simulink model "Kalman_modelling"  (R2020b)
settings: Solver=VariableStepAuto  StartTime=0.0  StopTime=10.0  RelTol=1e-3
values from neighbouring files (symbols this model uses):
  A_d = sys_d.A    [sample_ss.m]
  B_d = sys_d.B    [sample_ss.m]
  C_d = sys_d.C    [sample_ss.m]
  dT = 0.05    [sample_ss.m]
  G = eye(6)    [sample_ss.m]
  Qcov = diag(0.15*ones(1,size(A_m,1)))    [sample_ss.m]
  Rcov = diag(0.05*ones(1,size(A_m,1)))    [sample_ss.m]
undefined symbols (not defined in the file or in its folder): L
libraries: simulink x2
settings Model: Creator=surya  LastModifiedBy=surya

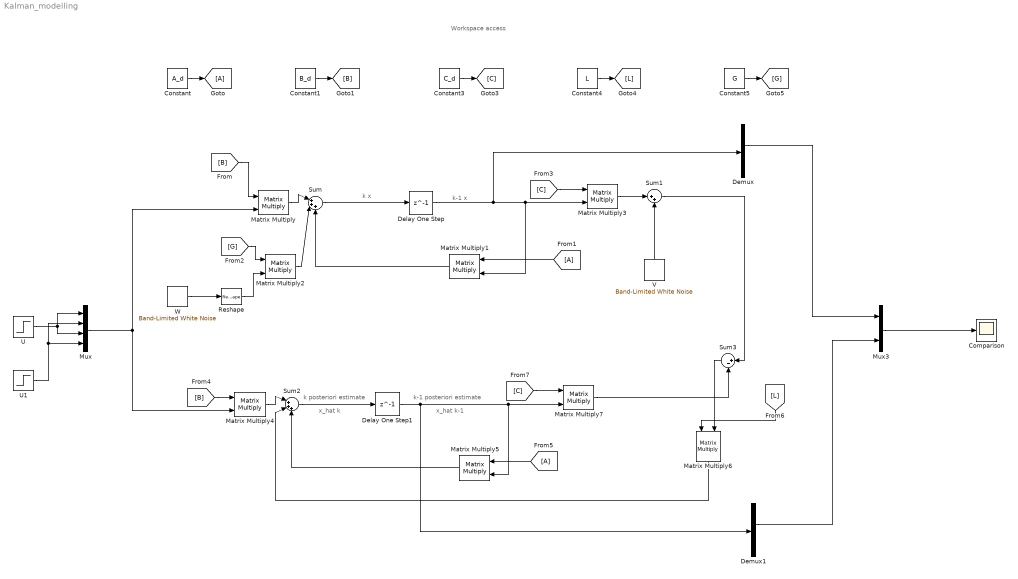
== system Kalman_modelling ==
  note: Workspace access
  note: x_hat k
  note: k x
  note: k-1 x
  note: k-1 posteriori estimate
  note: k posteriori estimate
  note: x_hat k-1
  Comparison : Scope
  Constant : Constant  Value=A_d
  Constant1 : Constant  Value=B_d
  Constant3 : Constant  Value=C_d
  Constant4 : Constant  Value=L
  Constant5 : Constant  Value=G
  Delay One Step : Delay  DelayLength=1  SampleTime=dT
  Delay One Step1 : Delay  DelayLength=1  SampleTime=dT
  Demux : Demux  Outputs=length(A_d)
  Demux1 : Demux  Outputs=length(A_d)
  Matrix Multiply{,1..7} (8 alike) : Product  Multiplication=Matrix(*)
  Mux : Mux
  Mux3 : Mux  Inputs=2
  Reshape : Reshape  OutputDimensionality=Customize  OutputDimensions=[length(G(1,:)),1]
  Sum : Sum  Inputs=|+++
  Sum1 : Sum  Inputs=|++
  Sum2 : Sum  Inputs=|+++
  Sum3 : Sum  Inputs=|+-
  U : Step  SampleTime=0
  U1 : Step  After=1/2  SampleTime=0
  V : simulink/Sources/Band-Limited White Noise  Cov=[Rcov(1)*dT Rcov(1)*dT Rcov(1)*dT Rcov(1)*dT Rcov(1)*dT Rcov(1)*dT]  Ts=dT  seed=[23341]
  W : simulink/Sources/Band-Limited White Noise  Cov=[Qcov(1)*dT Qcov(1)*dT Qcov(1)*dT Qcov(1)*dT Qcov(1)*dT Qcov(1)*dT]  Ts=dT  seed=[23341]
  wires:
  Constant/1 -> [A]
  Constant1/1 -> [B]
  Constant3/1 -> [C]
  Constant4/1 -> [L]
  Constant5/1 -> [G]
  U/1 -> Mux/3, Mux/1
  [B] -> Matrix Multiply/1
  Matrix Multiply/1 -> Sum/1
  Sum/1 -> Delay One Step/1
  Matrix Multiply1/1 -> Sum/3
  [C] -> Matrix Multiply3/1
  Matrix Multiply3/1 -> Sum1/1
  Sum1/1 -> Sum3/1
  Mux/1 -> Matrix Multiply4/2, Matrix Multiply/2
  Delay One Step1/1 -> Demux1/1, Matrix Multiply5/2, Matrix Multiply7/2
  [C] -> Matrix Multiply7/1
  Matrix Multiply4/1 -> Sum2/1
  [B] -> Matrix Multiply4/1
  Matrix Multiply7/1 -> Sum3/2
  Matrix Multiply6/1 -> Sum2/2
  Matrix Multiply5/1 -> Sum2/3
  Sum2/1 -> Delay One Step1/1
  Mux3/1 -> Comparison/1
  [G] -> Matrix Multiply2/1
  Reshape/1 -> Matrix Multiply2/2
  Matrix Multiply2/1 -> Sum/2
  Delay One Step/1 -> Demux/1, Matrix Multiply1/2, Matrix Multiply3/2
  [A] -> Matrix Multiply1/1
  W/1 -> Reshape/1
  V/1 -> Sum1/2
  [L] -> Matrix Multiply6/1
  Sum3/1 -> Matrix Multiply6/2
  [A] -> Matrix Multiply5/1
  U1/1 -> Mux/4, Mux/2
  Demux/3 -> Mux3/1
  Demux1/3 -> Mux3/2
